simulink model "SIMULINK_InvertedPendulum_PDC"  (R2020a)
settings: Solver=FixedStepAuto  StartTime=0.0  StopTime=30  FixedStep=0.001  RelTol=1e-3
settings Model: Creator=CepaTech  LastModifiedBy=CepaTech

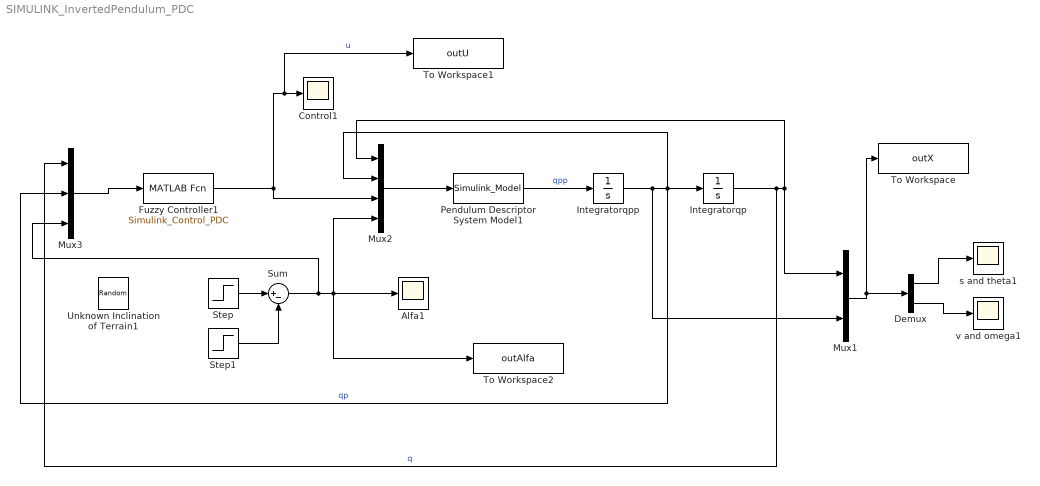
== system SIMULINK_InvertedPendulum_PDC ==
  Alfa1 : Scope
  Control1 : Scope
  Demux : Demux  Outputs=2
  Fuzzy Controller1 : MATLABFcn  MATLABFcn=Simulink_Control_PDC
  Integratorqp : Integrator  InitialCondition=[0 0]
  Integratorqpp : Integrator  InitialCondition=[0 0.785398163397448]
  Mux1 : Mux  Inputs=2
  Mux2 : Mux
  Mux3 : Mux  Inputs=3
  Pendulum Descriptor System Model1 : MATLABFcn  MATLABFcn=Simulink_Model
  Step : Step  Time=10  After=deg2rad(6)  SampleTime=0
  Step1 : Step  Time=20  After=deg2rad(6)  SampleTime=0
  Sum : Sum  Inputs=|+-
  To Workspace : ToWorkspace  VariableName=outX  SampleTime=-1
  To Workspace1 : ToWorkspace  VariableName=outU  SampleTime=-1
  To Workspace2 : ToWorkspace  VariableName=outAlfa  SampleTime=-1
  Unknown Inclination of Terrain1 : UniformRandomNumber  Minimum=-deg2rad(10)  Maximum=deg2rad(10)  SampleTime=0.5
  s and theta1 : Scope
  v and omega1 : Scope
  wires:
  Demux/1 -> s and theta1/1
  Demux/2 -> v and omega1/1
  Fuzzy Controller1/1 -> To Workspace1/1, Control1/1, Mux2/3  "u"
  Pendulum Descriptor System Model1/1 -> Integratorqpp/1  "qpp"
  Mux3/1 -> Fuzzy Controller1/1
  Mux2/1 -> Pendulum Descriptor System Model1/1
  Integratorqpp/1 -> Mux1/2, Mux2/2, Mux3/2, Integratorqp/1  "qp"
  Integratorqp/1 -> Mux3/1, Mux1/1, Mux2/1  "q"
  Mux1/1 -> To Workspace/1, Demux/1
  Step/1 -> Sum/1
  Step1/1 -> Sum/2
  Sum/1 -> Mux3/3, To Workspace2/1, Alfa1/1, Mux2/4
